simulink subsystem "Coulomb_counting"  (R2019b)
settings: Solver=VariableStepAuto  StartTime=0.0  StopTime=10.0  RelTol=1e-3
settings Model: Creator=PcElettronicaDynamis  LastModifiedBy=PcElettronicaDynamis

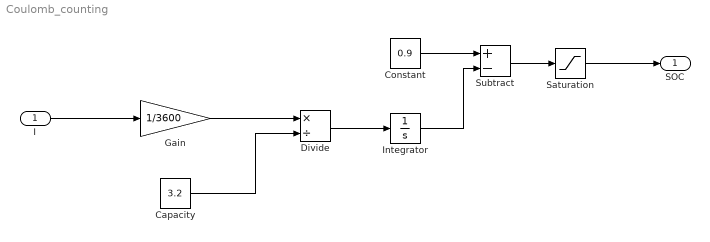
== system Coulomb_counting ==
  I : Inport
  Capacity : Constant  Value=3.2
  Constant : Constant  Value=0.9
  Divide : Product  Inputs=*/
  Gain : Gain  Gain=1/3600
  Integrator : Integrator
  Saturation : Saturate  UpperLimit=1  LowerLimit=0
  Subtract : Sum  Inputs=+-
  SOC : Outport  VectorParamsAs1DForOutWhenUnconnected=off
  wires:
  Capacity/1 -> Divide/2
  Divide/1 -> Integrator/1
  Constant/1 -> Subtract/1
  Subtract/1 -> Saturation/1
  Integrator/1 -> Subtract/2
  Saturation/1 -> SOC/1
  Gain/1 -> Divide/1
  I/1 -> Gain/1
